simulink model "ex_simulink_model2"  (R2022b)
settings: Solver=VariableStepAuto  StartTime=0.0  StopTime=100.0  RelTol=1e-3
settings Model: Creator=Daniel  LastModifiedBy=Dan
settings SolverCC: AlgebraicLoopSolver=TrustRegion
settings DebuggingCC: UnconnectedInputMsg=warning  UnconnectedOutputMsg=warning  UnconnectedLineMsg=warning  SFMachineParentedDataDiag=warning
settings ModelReferenceCC: EnableRefExpFcnMdlSchedulingChecks=on
settings RTWCC: DLArmComputeVersion=19.05

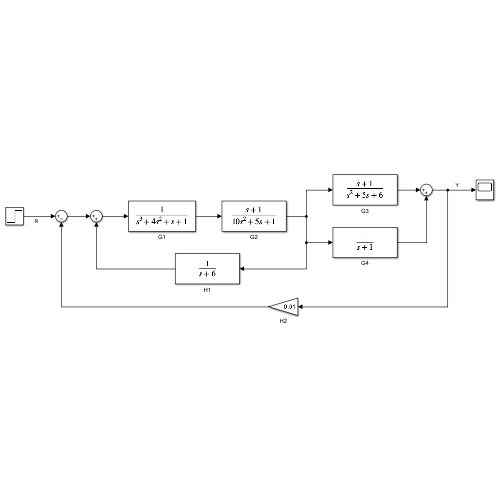
[thumbnail: Simulink's stored preview of the top-level diagram]
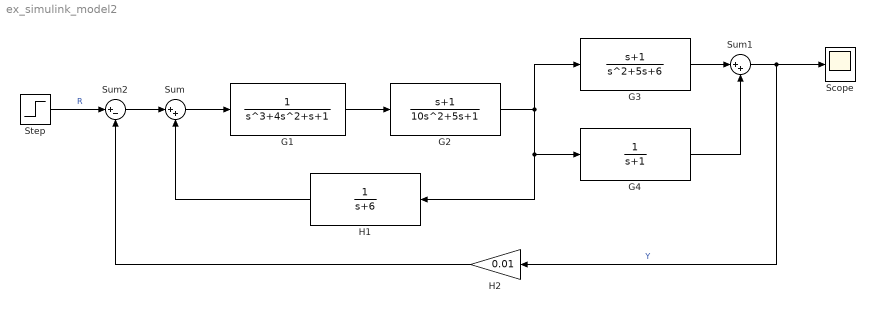
== system ex_simulink_model2 ==
  G1 : TransferFcn  Denominator=[1 4 1 1]
  G2 : TransferFcn  Numerator=[1 1]  Denominator=[10 5 1]
  G3 : TransferFcn  Numerator=[1 1]  Denominator=[1 5 6]
  G4 : TransferFcn  Denominator=[1 1]
  H1 : TransferFcn  Denominator=[1 6]
  H2 : Gain  Gain=0.01
  Scope : Scope
  Step : Step  SampleTime=0
  Sum : Sum  Inputs=|++
  Sum1 : Sum  Inputs=|++
  Sum2 : Sum  Inputs=|+-
  wires:
  G1/1 -> G2/1
  G2/1 -> G4/1, H1/1, G3/1
  G3/1 -> Sum1/1
  G4/1 -> Sum1/2
  Sum/1 -> G1/1
  Sum2/1 -> Sum/1
  H1/1 -> Sum/2
  H2/1 -> Sum2/2
  Sum1/1 -> Scope/1, H2/1  "Y"
  Step/1 -> Sum2/1  "R"
